simulink model "full_maneuver_single_veh"  (R2020a)
settings: Solver=VariableStepAuto  StartTime=0.0  StopTime=90  FixedStep=0.1  MaxStep=5e-2  RelTol=1e-3
InitFcn:
  | totalVehicles = 5;
  | if exist('vehStatesBus', 'var')==0
  | load vehBuses
  | end
  | if exist('vehErrorsBus', 'var')==0
  | load vehBuses
  | end
libraries: simulink x69, powerlib_meascontrol x6, autolibshared x6, dspsigops x3, eeGeneralControl x2
(part 3 of 6)

== system full_maneuver_single_veh/Fo/Regular Vehicle Following ==
  ego : Inport
  leader : Inport  Port=2
  leaderChange : Inport  Port=3
  extraSpaceFlag : Inport  Port=4
  Bus Selector : BusSelector  OutputSignals=u
  Compute Errors : Subsystem
  Constant : Constant  Value=0
  Define Desired Distance : Subsystem
  NOT : Logic  Operator=NOT  IconShape=distinctive  AllPortsSameDT=off  OutDataTypeStr=boolean
  Rate Limiter : RateLimiter  RisingSlewLimit=maxJerk  FallingSlewLimit=minJerk  SampleTimeMode=inherited
  Rate Limiter1 : RateLimiter  RisingSlewLimit=maxComfJerk  FallingSlewLimit=minComfJerk  SampleTimeMode=inherited
  Switch : Switch  Criteria=u2 > Threshold
  Switch1 : Switch  Criteria=u2 > Threshold
  Veh Following : Subsystem  TreatAsAtomicUnit=on
  Velocity Control : Subsystem  TreatAsAtomicUnit=on
  Velocity Error : Subsystem
  comf saturation : Saturate  UpperLimit=maxComfAccel  LowerLimit=minComfAccel
  errorScope : Scope
  freeFlowVel : Constant  Value=freeFlowVel
  safe saturation : Saturate  UpperLimit=maxAcceleration  LowerLimit=minAcceleration
  switch : Subsystem
  veh foll state : Scope  NumInputPorts=2
  u : Outport  VectorParamsAs1DForOutWhenUnconnected=off
  errors : Outport  Port=2  VectorParamsAs1DForOutWhenUnconnected=off
  gap : Outport  Port=3  VectorParamsAs1DForOutWhenUnconnected=off
  leaderInRange : Outport  Port=4  VectorParamsAs1DForOutWhenUnconnected=off
  wires:
  NOT/1 -> Velocity Error/3(inRange)
  Velocity Error/1(ev) -> Velocity Control/1(ev)
  Velocity Error/2(ea) -> Velocity Control/2(ea)
  leaderChange/1 -> Veh Following/4(leaderChange)
  Veh Following/1(u) -> Switch/1
  Constant/1 -> Compute Errors/5(velFilterReset)
  leader/1 -> Compute Errors/2(leader)
  switch/1(inRange) -> veh foll state/1, Switch/2, leaderInRange/1, Veh Following/5(inRange), NOT/1
  Compute Errors/1(errors) -> switch/1(errors), Veh Following/1(errors), errors/1, errorScope/1
  comf saturation/1 -> Rate Limiter1/1
  safe saturation/1 -> Rate Limiter/1
  Rate Limiter/1 -> Switch1/1  "sat(u)"
  Switch1/1 -> u/1
  Switch/1 -> veh foll state/2, safe saturation/1, comf saturation/1
  Rate Limiter1/1 -> Switch1/3  "sat(u)"
  Compute Errors/3("gap ") -> gap/1, switch/3(gap)
  ego/1 -> Compute Errors/1(ego), Bus Selector/1, Velocity Error/1(ego)
  Velocity Control/1(u) -> Switch/3
  freeFlowVel/1 -> Velocity Error/2(velRef), switch/6(vRef)
  Compute Errors/4(unsafeFlag) -> Switch1/2
  Bus Selector/1 -> Veh Following/3(realInput), Velocity Control/3(realInput)  "<u>"
  Compute Errors/2(errorsDot) -> switch/2(errorsDot), Veh Following/2(errorsDot)
  extraSpaceFlag/1 -> Define Desired Distance/1(extraSpaceFlag)
  Define Desired Distance/1(h) -> Compute Errors/3(h), switch/4(h)
  Define Desired Distance/2(d0) -> Compute Errors/4(d0), switch/5(d0)

== system full_maneuver_single_veh/Fo/findLeader ==
  ego : Inport
  all : Inport  Port=2
  lcFlag : Inport  Port=3
  state : Inport  Port=4
  Compare To Constant : simulink/Logic and Bit Operations/Compare To Constant  relop=~=  const=4  OutDataTypeStr=boolean
  Detect Change : simulink/Logic and Bit Operations/Detect Change  vinit=0  OutDataTypeStr=boolean
  NOT : Logic  Operator=NOT  IconShape=distinctive  AllPortsSameDT=off  OutDataTypeStr=boolean
  OR : Logic  Operator=OR  IconShape=distinctive  AllPortsSameDT=off  OutDataTypeStr=boolean
  Selector : Selector  InputPortWidth=totalVehicles+1  IndexOptions=Index vector (port)  Indices=[1]  OutputSizes=1
  Subsystem : Subsystem
  Vector Concatenate : Concatenate
  farAwayVeh : Subsystem
  realLeaderIdx : Scope
  leader : Outport  VectorParamsAs1DForOutWhenUnconnected=off
  leaderChange : Outport  Port=2  InitialOutput=1  VectorParamsAs1DForOutWhenUnconnected=off
  wires:
  Compare To Constant/1 -> OR/2
  state/1 -> Compare To Constant/1
  ego/1 -> farAwayVeh/1(ego), Subsystem/1(ego)
  all/1 -> Vector Concatenate/1, Subsystem/2(all)
  Subsystem/1(idx) -> realLeaderIdx/1, Selector/2, Detect Change/1
  OR/1 -> Subsystem/Enable
  lcFlag/1 -> NOT/1
  NOT/1 -> OR/1
  Selector/1 -> leader/1
  farAwayVeh/1(Out1) -> Vector Concatenate/2
  Vector Concatenate/1 -> Selector/1
  Detect Change/1 -> leaderChange/1

== system full_maneuver_single_veh/Fo/states routing ==
  delta : Inport
  Info : Inport  Port=2
  u : Inport  Port=3
  Bus Creator : BusCreator  Inputs=7  OutDataTypeStr=Bus: vehStatesBus  NonVirtualBus=on
      settings: InheritFromInputs=off
  Bus Selector : BusSelector  OutputSignals=BdyFrm.Cg.Vel.ydot,BdyFrm.Cg.AngVel.r,InertFrm.RearAxl.Disp.X,InertFrm.Cg.Disp.Y,InertFrm.RearAxl.Vel.Xdot,BdyFrm.Cg.Acc.xddot,InertFrm.Cg.Ang.psi
  Mux : Mux
  latStates : Outport
  observedStates : Outport  Port=2
  wires:
  Bus Creator/1 -> observedStates/1
  Bus Selector/2 -> Mux/4  "<r>"
  Bus Selector/1 -> Mux/2  "<ydot>"
  Mux/1 -> latStates/1
  delta/1 -> Bus Creator/7
  u/1 -> Bus Creator/6  "u"
  Bus Selector/7 -> Mux/3, Bus Creator/5  "<psi>"
  Bus Selector/6 -> Bus Creator/4  "<xddot>"
  Bus Selector/5 -> Bus Creator/3  "<Xdot>"
  Bus Selector/4 -> Mux/1, Bus Creator/2  "<Y>"
  Bus Selector/3 -> Bus Creator/1  "<X>"
  Info/1 -> Bus Selector/1

== system full_maneuver_single_veh/Ld/Regular Vehicle Following ==
  ego : Inport
  leader : Inport  Port=2
  leaderChange : Inport  Port=3
  extraSpaceFlag : Inport  Port=4
  Bus Selector : BusSelector  OutputSignals=u
  Compute Errors : Subsystem
  Constant : Constant  Value=0
  Define Desired Distance : Subsystem
  NOT : Logic  Operator=NOT  IconShape=distinctive  AllPortsSameDT=off  OutDataTypeStr=boolean
  Rate Limiter : RateLimiter  RisingSlewLimit=maxJerk  FallingSlewLimit=minJerk  SampleTimeMode=inherited
  Rate Limiter1 : RateLimiter  RisingSlewLimit=maxComfJerk  FallingSlewLimit=minComfJerk  SampleTimeMode=inherited
  Switch : Switch  Criteria=u2 > Threshold
  Switch1 : Switch  Criteria=u2 > Threshold
  Veh Following : Subsystem  TreatAsAtomicUnit=on
  Velocity Control : Subsystem  TreatAsAtomicUnit=on
  Velocity Error : Subsystem
  comf saturation : Saturate  UpperLimit=maxComfAccel  LowerLimit=minComfAccel
  errorScope : Scope
  freeFlowVel : Constant  Value=freeFlowVel
  safe saturation : Saturate  UpperLimit=maxAcceleration  LowerLimit=minAcceleration
  switch : Subsystem
  veh foll state : Scope  NumInputPorts=2
  u : Outport  VectorParamsAs1DForOutWhenUnconnected=off
  errors : Outport  Port=2  VectorParamsAs1DForOutWhenUnconnected=off
  gap : Outport  Port=3  VectorParamsAs1DForOutWhenUnconnected=off
  leaderInRange : Outport  Port=4  VectorParamsAs1DForOutWhenUnconnected=off
  wires:
  NOT/1 -> Velocity Error/3(inRange)
  Velocity Error/1(ev) -> Velocity Control/1(ev)
  Velocity Error/2(ea) -> Velocity Control/2(ea)
  leaderChange/1 -> Veh Following/4(leaderChange)
  Veh Following/1(u) -> Switch/1
  Constant/1 -> Compute Errors/5(velFilterReset)
  leader/1 -> Compute Errors/2(leader)
  switch/1(inRange) -> veh foll state/1, Switch/2, leaderInRange/1, Veh Following/5(inRange), NOT/1
  Compute Errors/1(errors) -> switch/1(errors), Veh Following/1(errors), errors/1, errorScope/1
  comf saturation/1 -> Rate Limiter1/1
  safe saturation/1 -> Rate Limiter/1
  Rate Limiter/1 -> Switch1/1  "sat(u)"
  Switch1/1 -> u/1
  Switch/1 -> veh foll state/2, safe saturation/1, comf saturation/1
  Rate Limiter1/1 -> Switch1/3  "sat(u)"
  Compute Errors/3("gap ") -> gap/1, switch/3(gap)
  ego/1 -> Compute Errors/1(ego), Bus Selector/1, Velocity Error/1(ego)
  Velocity Control/1(u) -> Switch/3
  freeFlowVel/1 -> Velocity Error/2(velRef), switch/6(vRef)
  Compute Errors/4(unsafeFlag) -> Switch1/2
  Bus Selector/1 -> Veh Following/3(realInput), Velocity Control/3(realInput)  "<u>"
  Compute Errors/2(errorsDot) -> switch/2(errorsDot), Veh Following/2(errorsDot)
  extraSpaceFlag/1 -> Define Desired Distance/1(extraSpaceFlag)
  Define Desired Distance/1(h) -> Compute Errors/3(h), switch/4(h)
  Define Desired Distance/2(d0) -> Compute Errors/4(d0), switch/5(d0)

== system full_maneuver_single_veh/Ld/findLeader ==
  ego : Inport
  all : Inport  Port=2
  lcFlag : Inport  Port=3
  state : Inport  Port=4
  Compare To Constant : simulink/Logic and Bit Operations/Compare To Constant  relop=~=  const=4  OutDataTypeStr=boolean
  Detect Change : simulink/Logic and Bit Operations/Detect Change  vinit=0  OutDataTypeStr=boolean
  NOT : Logic  Operator=NOT  IconShape=distinctive  AllPortsSameDT=off  OutDataTypeStr=boolean
  OR : Logic  Operator=OR  IconShape=distinctive  AllPortsSameDT=off  OutDataTypeStr=boolean
  Selector : Selector  InputPortWidth=totalVehicles+1  IndexOptions=Index vector (port)  Indices=[1]  OutputSizes=1
  Subsystem : Subsystem
  Vector Concatenate : Concatenate
  farAwayVeh : Subsystem
  realLeaderIdx : Scope
  leader : Outport  VectorParamsAs1DForOutWhenUnconnected=off
  leaderChange : Outport  Port=2  InitialOutput=1  VectorParamsAs1DForOutWhenUnconnected=off
  wires:
  Compare To Constant/1 -> OR/2
  state/1 -> Compare To Constant/1
  ego/1 -> farAwayVeh/1(ego), Subsystem/1(ego)
  all/1 -> Vector Concatenate/1, Subsystem/2(all)
  Subsystem/1(idx) -> realLeaderIdx/1, Selector/2, Detect Change/1
  OR/1 -> Subsystem/Enable
  lcFlag/1 -> NOT/1
  NOT/1 -> OR/1
  Selector/1 -> leader/1
  farAwayVeh/1(Out1) -> Vector Concatenate/2
  Vector Concatenate/1 -> Selector/1
  Detect Change/1 -> leaderChange/1

== system full_maneuver_single_veh/Ld/states routing ==
  delta : Inport
  Info : Inport  Port=2
  u : Inport  Port=3
  Bus Creator : BusCreator  Inputs=7  OutDataTypeStr=Bus: vehStatesBus  NonVirtualBus=on
      settings: InheritFromInputs=off
  Bus Selector : BusSelector  OutputSignals=BdyFrm.Cg.Vel.ydot,BdyFrm.Cg.AngVel.r,InertFrm.RearAxl.Disp.X,InertFrm.Cg.Disp.Y,InertFrm.RearAxl.Vel.Xdot,BdyFrm.Cg.Acc.xddot,InertFrm.Cg.Ang.psi
  Mux : Mux
  latStates : Outport
  observedStates : Outport  Port=2
  wires:
  Bus Creator/1 -> observedStates/1
  Bus Selector/2 -> Mux/4  "<r>"
  Bus Selector/1 -> Mux/2  "<ydot>"
  Mux/1 -> latStates/1
  delta/1 -> Bus Creator/7
  u/1 -> Bus Creator/6  "u"
  Bus Selector/7 -> Mux/3, Bus Creator/5  "<psi>"
  Bus Selector/6 -> Bus Creator/4  "<xddot>"
  Bus Selector/5 -> Bus Creator/3  "<Xdot>"
  Bus Selector/4 -> Mux/1, Bus Creator/2  "<Y>"
  Bus Selector/3 -> Bus Creator/1  "<X>"
  Info/1 -> Bus Selector/1

== system full_maneuver_single_veh/Lo/Regular Vehicle Following ==
  ego : Inport
  leader : Inport  Port=2
  leaderChange : Inport  Port=3
  extraSpaceFlag : Inport  Port=4
  Bus Selector : BusSelector  OutputSignals=u
  Compute Errors : Subsystem
  Constant : Constant  Value=0
  Define Desired Distance : Subsystem
  NOT : Logic  Operator=NOT  IconShape=distinctive  AllPortsSameDT=off  OutDataTypeStr=boolean
  Rate Limiter : RateLimiter  RisingSlewLimit=maxJerk  FallingSlewLimit=minJerk  SampleTimeMode=inherited
  Rate Limiter1 : RateLimiter  RisingSlewLimit=maxComfJerk  FallingSlewLimit=minComfJerk  SampleTimeMode=inherited
  Switch : Switch  Criteria=u2 > Threshold
  Switch1 : Switch  Criteria=u2 > Threshold
  Veh Following : Subsystem  TreatAsAtomicUnit=on
  Velocity Control : Subsystem  TreatAsAtomicUnit=on
  Velocity Error : Subsystem
  comf saturation : Saturate  UpperLimit=maxComfAccel  LowerLimit=minComfAccel
  errorScope : Scope
  freeFlowVel : Constant  Value=freeFlowVel
  safe saturation : Saturate  UpperLimit=maxAcceleration  LowerLimit=minAcceleration
  switch : Subsystem
  veh foll state : Scope  NumInputPorts=2
  u : Outport  VectorParamsAs1DForOutWhenUnconnected=off
  errors : Outport  Port=2  VectorParamsAs1DForOutWhenUnconnected=off
  gap : Outport  Port=3  VectorParamsAs1DForOutWhenUnconnected=off
  leaderInRange : Outport  Port=4  VectorParamsAs1DForOutWhenUnconnected=off
  wires:
  Define Desired Distance/2(d0) -> switch/5(d0), Compute Errors/4(d0)
  Define Desired Distance/1(h) -> switch/4(h), Compute Errors/3(h)
  extraSpaceFlag/1 -> Define Desired Distance/1(extraSpaceFlag)
  Compute Errors/2(errorsDot) -> Veh Following/2(errorsDot), switch/2(errorsDot)
  Bus Selector/1 -> Velocity Control/3(realInput), Veh Following/3(realInput)  "<u>"
  Compute Errors/4(unsafeFlag) -> Switch1/2
  freeFlowVel/1 -> switch/6(vRef), Velocity Error/2(velRef)
  Velocity Control/1(u) -> Switch/3
  ego/1 -> Velocity Error/1(ego), Bus Selector/1, Compute Errors/1(ego)
  Compute Errors/3("gap ") -> switch/3(gap), gap/1
  Rate Limiter1/1 -> Switch1/3  "sat(u)"
  Switch/1 -> comf saturation/1, safe saturation/1, veh foll state/2
  Switch1/1 -> u/1
  Rate Limiter/1 -> Switch1/1  "sat(u)"
  safe saturation/1 -> Rate Limiter/1
  comf saturation/1 -> Rate Limiter1/1
  Compute Errors/1(errors) -> errorScope/1, errors/1, Veh Following/1(errors), switch/1(errors)
  switch/1(inRange) -> NOT/1, Veh Following/5(inRange), leaderInRange/1, Switch/2, veh foll state/1
  leader/1 -> Compute Errors/2(leader)
  Constant/1 -> Compute Errors/5(velFilterReset)
  Veh Following/1(u) -> Switch/1
  leaderChange/1 -> Veh Following/4(leaderChange)
  Velocity Error/2(ea) -> Velocity Control/2(ea)
  Velocity Error/1(ev) -> Velocity Control/1(ev)
  NOT/1 -> Velocity Error/3(inRange)

== system full_maneuver_single_veh/Lo/findLeader ==
  ego : Inport
  all : Inport  Port=2
  lcFlag : Inport  Port=3
  state : Inport  Port=4
  Compare To Constant : simulink/Logic and Bit Operations/Compare To Constant  relop=~=  const=4  OutDataTypeStr=boolean
  Detect Change : simulink/Logic and Bit Operations/Detect Change  vinit=0  OutDataTypeStr=boolean
  NOT : Logic  Operator=NOT  IconShape=distinctive  AllPortsSameDT=off  OutDataTypeStr=boolean
  OR : Logic  Operator=OR  IconShape=distinctive  AllPortsSameDT=off  OutDataTypeStr=boolean
  Selector : Selector  InputPortWidth=totalVehicles+1  IndexOptions=Index vector (port)  Indices=[1]  OutputSizes=1
  Subsystem : Subsystem
  Vector Concatenate : Concatenate
  farAwayVeh : Subsystem
  realLeaderIdx : Scope
  leader : Outport  VectorParamsAs1DForOutWhenUnconnected=off
  leaderChange : Outport  Port=2  InitialOutput=1  VectorParamsAs1DForOutWhenUnconnected=off
  wires:
  Detect Change/1 -> leaderChange/1
  Vector Concatenate/1 -> Selector/1
  farAwayVeh/1(Out1) -> Vector Concatenate/2
  Selector/1 -> leader/1
  NOT/1 -> OR/1
  lcFlag/1 -> NOT/1
  OR/1 -> Subsystem/Enable
  Subsystem/1(idx) -> Detect Change/1, Selector/2, realLeaderIdx/1
  all/1 -> Subsystem/2(all), Vector Concatenate/1
  ego/1 -> Subsystem/1(ego), farAwayVeh/1(ego)
  state/1 -> Compare To Constant/1
  Compare To Constant/1 -> OR/2

== system full_maneuver_single_veh/Lo/states routing ==
  delta : Inport
  Info : Inport  Port=2
  u : Inport  Port=3
  Bus Creator : BusCreator  Inputs=7  OutDataTypeStr=Bus: vehStatesBus  NonVirtualBus=on
      settings: InheritFromInputs=off
  Bus Selector : BusSelector  OutputSignals=BdyFrm.Cg.Vel.ydot,BdyFrm.Cg.AngVel.r,InertFrm.RearAxl.Disp.X,InertFrm.Cg.Disp.Y,InertFrm.RearAxl.Vel.Xdot,BdyFrm.Cg.Acc.xddot,InertFrm.Cg.Ang.psi
  Mux : Mux
  latStates : Outport
  observedStates : Outport  Port=2
  wires:
  Info/1 -> Bus Selector/1
  Bus Selector/3 -> Bus Creator/1  "<X>"
  Bus Selector/4 -> Bus Creator/2, Mux/1  "<Y>"
  Bus Selector/5 -> Bus Creator/3  "<Xdot>"
  Bus Selector/6 -> Bus Creator/4  "<xddot>"
  Bus Selector/7 -> Bus Creator/5, Mux/3  "<psi>"
  u/1 -> Bus Creator/6  "u"
  delta/1 -> Bus Creator/7
  Mux/1 -> latStates/1
  Bus Selector/1 -> Mux/2  "<ydot>"
  Bus Selector/2 -> Mux/4  "<r>"
  Bus Creator/1 -> observedStates/1

== system full_maneuver_single_veh/p1/Error to Follower ==
  ego : Inport
  follower : Inport  Port=2
  Bus Selector : BusSelector  OutputSignals=X,Xdot
  Bus Selector1 : BusSelector  OutputSignals=X,Xdot
  Multiply : Product
  Mux : Mux  Inputs=2
  Sum : Sum  Inputs=-+|
  Sum1 : Sum  Inputs=++|
  Sum2 : Sum  Inputs=+-|
  Sum3 : Sum  Inputs=|++
  Sum4 : Sum  Inputs=-+|
  d0 : Constant  Value=d0
  h : Constant  Value=h
  vLen : Constant  Value=lr+lf
  errors : Outport  VectorParamsAs1DForOutWhenUnconnected=off
  wires:
  Mux/1 -> errors/1
  Sum4/1 -> Mux/2
  Bus Selector1/2 -> Sum4/2  "<Xdot>"
  Bus Selector/2 -> Multiply/1, Sum4/1  "<Xdot>"
  ego/1 -> Bus Selector1/1
  follower/1 -> Bus Selector/1
  vLen/1 -> Sum1/1
  Multiply/1 -> Sum3/1
  Sum/1 -> Sum2/1  "gap"
  Bus Selector/1 -> Sum1/2  "<X>"
  Sum3/1 -> Sum2/2  "desired  gap"
  Sum1/1 -> Sum/1  "x (front bumber)"
  Bus Selector1/1 -> Sum/2  "<X>"
  Sum2/1 -> Mux/1
  h/1 -> Multiply/2  "time headway"
  d0/1 -> Sum3/2  "gap at  standstill"

== system full_maneuver_single_veh/p1/Find Leader ==
  ego : Inport
  all : Inport  Port=2
  lcFlag : Inport  Port=3
  state : Inport  Port=4
  Compare To Constant : simulink/Logic and Bit Operations/Compare To Constant  relop=~=  const=4  OutDataTypeStr=boolean
  Detect Change : simulink/Logic and Bit Operations/Detect Change  vinit=0  OutDataTypeStr=boolean
  NOT : Logic  Operator=NOT  IconShape=distinctive  AllPortsSameDT=off  OutDataTypeStr=boolean
  OR : Logic  Operator=OR  IconShape=distinctive  AllPortsSameDT=off  OutDataTypeStr=boolean
  Selector : Selector  InputPortWidth=totalVehicles+1  IndexOptions=Index vector (port)  Indices=[1]  OutputSizes=1
  Subsystem : Subsystem
  Vector Concatenate : Concatenate
  farAwayVeh : Subsystem
  realLeaderIdx : Scope
  leader : Outport  VectorParamsAs1DForOutWhenUnconnected=off
  leaderChange : Outport  Port=2  InitialOutput=1  VectorParamsAs1DForOutWhenUnconnected=off
  wires:
  Detect Change/1 -> leaderChange/1
  Vector Concatenate/1 -> Selector/1
  farAwayVeh/1(Out1) -> Vector Concatenate/2
  Selector/1 -> leader/1
  NOT/1 -> OR/1
  lcFlag/1 -> NOT/1
  OR/1 -> Subsystem/Enable
  Subsystem/1(idx) -> Detect Change/1, Selector/2, realLeaderIdx/1
  all/1 -> Subsystem/2(all), Vector Concatenate/1
  ego/1 -> farAwayVeh/1(ego), Subsystem/1(ego)
  state/1 -> Compare To Constant/1
  Compare To Constant/1 -> OR/2

== system full_maneuver_single_veh/p1/Lateral Control ==
  measuredStates : Inport
  yRef : Inport  Port=2
  Enable : EnablePort
  Demux2 : Demux
  Full State Observer : Subsystem  Commented=on
  Gain : Gain  Gain=5
  Gain1 : Gain  Gain=Klat  Multiplication=Matrix(K*u)
  Integrator : Integrator  InitialCondition=y0
  Pad : dspsigops/Pad  padAlong=Columns  dimsToPad=1  valSrc=Specify via dialog  padVal=0  spec=Output size  padNumOutRowsSpecMethod=User-specified  numOutRows=4  padNumOutColsSpecMethod=User-specified  numOutCols=1  isVarDimsMode=off  padBeginning=0  padEnd=0  outSizeMode=User-specified  outSize=1  padSigAt=End  trunc_flag=None  roundingMode=Floor  overflowMode=off  truncOrWrapMode=Truncate  wrap_flag=None
      settings: SourceProductBaseCode=DS
  Rate Limiter : RateLimiter  RisingSlewLimit=maxDeltaDot  FallingSlewLimit=-maxDeltaDot  SampleTimeMode=inherited
  Saturation : Saturate  UpperLimit=maxDelta  LowerLimit=-maxDelta
  Saturation1 : Saturate  UpperLimit=2  LowerLimit=-2
  Scope : Scope  NumInputPorts=4
  Scope1 : Scope  NumInputPorts=2
  Selector : Selector  InputPortWidth=4  IndexOptions=Index vector (dialog)  Indices=[1]  OutputSizes=1
  Sum : Sum  Inputs=|+-
  Sum2 : Sum  Inputs=|+-
  delta : Outport  VectorParamsAs1DForOutWhenUnconnected=off
  ey : Outport  Port=2  VectorParamsAs1DForOutWhenUnconnected=off
  vy_hat : Outport  Port=3  InitialOutput=0.3  VectorParamsAs1DForOutWhenUnconnected=off
  wires:
  Rate Limiter/1 -> Full State Observer/2(delta), Scope1/1, delta/1  "delta"
  Demux2/1 -> Scope/1
  Integrator/1 -> Sum2/2, Pad/1
  Gain1/1 -> Scope1/2, Saturation/1
  Sum/1 -> Selector/1, Gain1/1
  Pad/1 -> Sum/1
  Demux2/4 -> Scope/4
  Demux2/2 -> vy_hat/1, Scope/2
  Sum2/1 -> Gain/1
  Saturation/1 -> Rate Limiter/1
  Demux2/3 -> Scope/3
  yRef/1 -> Sum2/1
  measuredStates/1 -> Full State Observer/1(measuredOutputs), Demux2/1, Sum/2  "estStates"
  Gain/1 -> Saturation1/1
  Saturation1/1 -> Integrator/1
  Selector/1 -> ey/1

== system full_maneuver_single_veh/p1/Maneuver State ==
  note: States are:
      | 0 - Lane keeping
      | 1 - Longitudinal Adjustment
      | 2 - Steady State
      | 3 - Safe to LC
      | 4 - Performing LC
      | 5 - LC is done
      | 6 - Long Adj done
  u : Inport
  errors : Inport  Port=2
  virtualErrors : Inport  Port=3
  followerErrors : Inport  Port=4
  canStartLC : Inport  Port=5
  extraSpace : Inport  Port=6
  lcDone : Inport  Port=7
  Enable : EnablePort
  AND : Logic  IconShape=distinctive  AllPortsSameDT=off  OutDataTypeStr=boolean
  AND1 : Logic  IconShape=distinctive  AllPortsSameDT=off  OutDataTypeStr=boolean
  AND2 : Logic  Inputs=3  IconShape=distinctive  AllPortsSameDT=off  OutDataTypeStr=boolean
  AND{3..7} (5 alike) : Logic  IconShape=distinctive  AllPortsSameDT=off  OutDataTypeStr=fixdt(1,16)
  Constant : Constant
  Data Type Conversion : DataTypeConversion  OutMin=0  OutMax=1  OutDataTypeStr=fixdt(1,16)
  Memory : Memory
  NOT1 : Logic  Operator=NOT  IconShape=distinctive  AllPortsSameDT=off  OutDataTypeStr=boolean
  On Delay : powerlib_meascontrol/Logic/On Delay  DelayType=On delay  delay=1  ic=0  Ts=0
  On Delay1 : powerlib_meascontrol/Logic/On Delay  DelayType=On delay  delay=0.2  ic=0  Ts=0
  Scope : Scope  NumInputPorts=5
  Sum : Sum  Inputs=++++++
  Triggered Subsystem : Subsystem  TreatAsAtomicUnit=on
  Triggered Subsystem1 : Subsystem  TreatAsAtomicUnit=on
  safeErrors : Subsystem
  safeErrors1 : Subsystem
  safeErrors2 : Subsystem
  steadyState : Subsystem
  state : Outport  InitialOutput=0  VectorParamsAs1DForOutWhenUnconnected=off
  wires:
  Memory/1 -> AND3/2
  AND4/1 -> AND5/1, Scope/2, Sum/3
  safeErrors/1(safetyFlag) -> AND4/2
  Sum/1 -> state/1
  AND3/1 -> AND4/1, Scope/1, Sum/2
  AND5/1 -> AND6/1, Scope/3, Sum/4
  Constant/1 -> Data Type Conversion/1, AND3/1
  AND6/1 -> Scope/4, Sum/5, AND7/1
  AND/1 -> AND7/2
  Data Type Conversion/1 -> Sum/1
  AND7/1 -> Triggered Subsystem/Trigger, Scope/5
  lcDone/1 -> AND6/2
  canStartLC/1 -> AND5/2
  Triggered Subsystem/1(Out1) -> Sum/6
  virtualErrors/1 -> safeErrors2/1(errors)
  errors/1 -> safeErrors1/1(errors)
  followerErrors/1 -> safeErrors/1(errors)
  On Delay1/1 -> AND/2
  AND2/1 -> Triggered Subsystem1/Trigger
  safeErrors1/1(safetyFlag) -> AND1/2
  extraSpace/1 -> NOT1/1, On Delay/1
  On Delay/1 -> AND2/3
  NOT1/1 -> On Delay1/1
  Triggered Subsystem1/1(Out1) -> Memory/1
  safeErrors2/1(safetyFlag) -> AND2/2
  steadyState/1(ssFlag) -> AND1/1
  AND1/1 -> AND2/1, AND/1  "steady state"
  u/1 -> steadyState/1(u)

== system full_maneuver_single_veh/p1/Platoon Gap Generation Management ==
  posInPlatoon : Inport
  strategy : Inport  Port=2
  platoonState : Inport  Port=3
  Enable : EnablePort
  Scope : Scope  NumInputPorts=2
  assignExtraSpace : MATLAB Function  TreatAsAtomicUnit=on
  assignvirtualLeader : MATLAB Function  TreatAsAtomicUnit=on
  assignVL : Outport  VectorParamsAs1DForOutWhenUnconnected=off
  extraSpace : Outport  Port=2  VectorParamsAs1DForOutWhenUnconnected=off
  wires:
  assignExtraSpace/1(extraSpaceFlag) -> Scope/2, extraSpace/1
  strategy/1 -> assignvirtualLeader/1(strategy), assignExtraSpace/1(strategy)
  posInPlatoon/1 -> assignvirtualLeader/2(posInPlatoon), assignExtraSpace/2(posInPlatoon)
  platoonState/1 -> assignvirtualLeader/3(platoonState), assignExtraSpace/3(platoonState)
  assignvirtualLeader/1(virtualLeaderFlag) -> Scope/1, assignVL/1

== system full_maneuver_single_veh/p1/Platoon LC Management ==
  platoonStates : Inport
  strategy : Inport  Port=2
  Compare To Constant : simulink/Logic and Bit Operations/Compare To Constant  relop=>  const=1  OutDataTypeStr=boolean
  Compare To Constant1 : simulink/Logic and Bit Operations/Compare To Constant  relop=>  const=2  OutDataTypeStr=boolean
  OR : Logic  Operator=OR  IconShape=distinctive  AllPortsSameDT=off  OutDataTypeStr=boolean
  Selector : Selector  IndexOptions=Index vector (port)  Indices=[1 3]  OutputSizes=1
  Width : Width
  Out1 : Outport  VectorParamsAs1DForOutWhenUnconnected=off
  wires:
  strategy/1 -> Compare To Constant/1
  Compare To Constant/1 -> OR/2
  OR/1 -> Out1/1
  platoonStates/1 -> Width/1, Selector/1
  Width/1 -> Selector/2
  Selector/1 -> Compare To Constant1/1
  Compare To Constant1/1 -> OR/1

== system full_maneuver_single_veh/p1/Regular Vehicle Following ==
  ego : Inport
  leader : Inport  Port=2
  leaderChange : Inport  Port=3
  extraSpaceFlag : Inport  Port=4
  Bus Selector : BusSelector  OutputSignals=u
  Compute Errors : Subsystem
  Constant : Constant  Value=0
  Define Desired Distance : Subsystem
  Rate Limiter : RateLimiter  RisingSlewLimit=maxJerk  FallingSlewLimit=minJerk  SampleTimeMode=inherited
  Rate Limiter1 : RateLimiter  RisingSlewLimit=maxComfJerk  FallingSlewLimit=minComfJerk  SampleTimeMode=inherited
  Switch : Switch  Criteria=u2 > Threshold
  Switch1 : Switch  Criteria=u2 > Threshold
  Veh Following : Subsystem  TreatAsAtomicUnit=on
  Velocity Control : Subsystem  TreatAsAtomicUnit=on
  Velocity Error : Subsystem
  comf saturation : Saturate  UpperLimit=maxComfAccel  LowerLimit=minComfAccel
  errorScope : Scope
  freeFlowVel : Constant  Value=freeFlowVel
  safe saturation : Saturate  UpperLimit=maxAcceleration  LowerLimit=minAcceleration
  switch free flow : Subsystem
  veh foll state : Scope  NumInputPorts=2
  u : Outport  VectorParamsAs1DForOutWhenUnconnected=off
  errors : Outport  Port=2  VectorParamsAs1DForOutWhenUnconnected=off
  gap : Outport  Port=3  VectorParamsAs1DForOutWhenUnconnected=off
  wires:
  Define Desired Distance/2(d0) -> switch free flow/5(d0), Compute Errors/4(d0)
  Define Desired Distance/1(h) -> switch free flow/4(h), Compute Errors/3(h)
  Compute Errors/2(errorsDot) -> switch free flow/2(errorsDot), Veh Following/2(errorsDot)
  Bus Selector/1 -> Velocity Control/3(realInput), Veh Following/3(realInput)  "<u>"
  Compute Errors/4(unsafeFlag) -> Switch1/2
  freeFlowVel/1 -> switch free flow/6(vRef), Velocity Error/2(velRef)
  Velocity Control/1(u) -> Switch/3
  ego/1 -> Velocity Error/1(ego), Bus Selector/1, Compute Errors/1(ego)
  Compute Errors/3("gap ") -> switch free flow/3(gap), gap/1
  Rate Limiter1/1 -> Switch1/3  "sat(u)"
  Switch/1 -> comf saturation/1, safe saturation/1, veh foll state/2
  Switch1/1 -> u/1
  Rate Limiter/1 -> Switch1/1  "sat(u)"
  safe saturation/1 -> Rate Limiter/1
  comf saturation/1 -> Rate Limiter1/1
  Compute Errors/1(errors) -> errorScope/1, errors/1, Veh Following/1(errors), switch free flow/1(errors)
  leader/1 -> Compute Errors/2(leader)
  Constant/1 -> Compute Errors/5(velFilterReset)
  Veh Following/1(u) -> Switch/1
  leaderChange/1 -> Veh Following/4(leaderChange)
  Velocity Error/2(ea) -> Velocity Control/2(ea)
  Velocity Error/1(ev) -> Velocity Control/1(ev)
  switch free flow/1(inRange) -> Veh Following/5(inRange), veh foll state/1, Switch/2
  extraSpaceFlag/1 -> Velocity Error/3(filterReset), Define Desired Distance/1(extraSpaceFlag)

== system full_maneuver_single_veh/p1/Subsystem ==
  state : Inport
  u : Inport  Port=2
  Compare To Constant : simulink/Logic and Bit Operations/Compare To Constant  relop===  const=7  OutDataTypeStr=boolean
  Scope : Scope
  Switch1 : Switch  Criteria=u2 > Threshold
  comf saturation : Saturate  UpperLimit=maxComfAccel  LowerLimit=minComfAccel
  comf jerk : RateLimiter  RisingSlewLimit=maxComfJerk  FallingSlewLimit=minComfJerk  SampleTimeMode=inherited
  safe saturation : Saturate  UpperLimit=maxAcceleration  LowerLimit=minAcceleration
  safe jerk : RateLimiter  RisingSlewLimit=maxJerk  FallingSlewLimit=minJerk  SampleTimeMode=inherited
  sat(u) : Outport  VectorParamsAs1DForOutWhenUnconnected=off
  wires:
  Compare To Constant/1 -> Switch1/2
  Switch1/1 -> sat(u)/1, Scope/1
  comf jerk/1 -> Switch1/3
  u/1 -> safe saturation/1, comf saturation/1
  state/1 -> Compare To Constant/1
  comf saturation/1 -> comf jerk/1
  safe jerk/1 -> Switch1/1
  safe saturation/1 -> safe jerk/1

== system full_maneuver_single_veh/p1/Triggered Subsystem ==
  Trigger : TriggerPort  VariantControl=Variant
  Constant : Constant
  lcFlag : Outport  InitialOutput=0  VectorParamsAs1DForOutWhenUnconnected=off
  wires:
  Constant/1 -> lcFlag/1

== system full_maneuver_single_veh/p1/Virtual Follower Manager ==
  all : Inport
  posInPlatoon : Inport  Port=2
  lcStrategy : Inport  Port=3
  Enable : EnablePort
  Selector1 : Selector  InputPortWidth=totalVehicles  IndexOptions=Index vector (port)  Indices=[1]  OutputSizes=1
  Width : Width
  determineVirtualFollower : MATLAB Function  TreatAsAtomicUnit=on
  virtualFollower : Outport
  wires:
  Selector1/1 -> virtualFollower/1
  all/1 -> Width/1, Selector1/1
  posInPlatoon/1 -> determineVirtualFollower/2(posInPlatoon)
  determineVirtualFollower/1(virtualFollowerIdx) -> Selector1/2
  lcStrategy/1 -> determineVirtualFollower/3(lcStrategy)
  Width/1 -> determineVirtualFollower/1(nVehicles)

== system full_maneuver_single_veh/p1/Virtual Leader Manager ==
  all : Inport
  lcFlag : Inport  Port=2
  lcDone : Inport  Port=3
  posInPlatoon : Inport  Port=4
  lcStrategy : Inport  Port=5
  Detect Change : simulink/Logic and Bit Operations/Detect Change  vinit=0  OutDataTypeStr=boolean
  Selector : Selector  InputPortWidth=totalVehicles  IndexOptions=Index vector (port)  Indices=[1]  OutputSizes=1
  Width : Width
  determineVirtualLeader : MATLAB Function  TreatAsAtomicUnit=on
  virtualVehs : Scope
  virtualLeader : Outport  VectorParamsAs1DForOutWhenUnconnected=off
  leaderChange : Outport  Port=2  VectorParamsAs1DForOutWhenUnconnected=off
  wires:
  lcStrategy/1 -> determineVirtualLeader/5(lcStrategy)
  posInPlatoon/1 -> determineVirtualLeader/4(posInPlatoon)
  lcDone/1 -> determineVirtualLeader/3(lcDone)
  lcFlag/1 -> determineVirtualLeader/2(lcFlag)
  Width/1 -> determineVirtualLeader/1(nVehicles)
  determineVirtualLeader/1(virtualLeaderIdx) -> virtualVehs/1, Detect Change/1, Selector/2
  Detect Change/1 -> leaderChange/1
  Selector/1 -> virtualLeader/1
  all/1 -> Width/1, Selector/1

== system full_maneuver_single_veh/p1/Virtual Vehicle Following ==
  ego : Inport
  virtualLeader : Inport  Port=2
  leaderChange : Inport  Port=3
  extraSpaceFlag : Inport  Port=4
  Bus Selector : BusSelector  OutputSignals=u
  Compute Errors : Subsystem
  Define Desired Distance : Subsystem
  Min Velocity Control : Subsystem  TreatAsAtomicUnit=on
  Min Velocity Error : Subsystem
  NOT : Logic  Operator=NOT  IconShape=distinctive  AllPortsSameDT=off  OutDataTypeStr=boolean
  Scope : Scope  NumInputPorts=2
  Switch : Switch  Criteria=u2 > Threshold
  Terminator : Terminator
  Virtual Leader Following : Subsystem  TreatAsAtomicUnit=on
  switch min vel : Subsystem
  vMin : Constant  Value=vMin
  u : Outport  InitialOutput=0  VectorParamsAs1DForOutWhenUnconnected=off
  virtualErrors : Outport  Port=2  OutputWhenDisabled=reset  InitialOutput=[0, 0]  VectorParamsAs1DForOutWhenUnconnected=off
  virtualGap : Outport  Port=3  OutputWhenDisabled=reset  InitialOutput=[0]  VectorParamsAs1DForOutWhenUnconnected=off
  wires:
  Define Desired Distance/2(d0) -> Compute Errors/4(d0), switch min vel/5(d0)
  Define Desired Distance/1(h) -> Compute Errors/3(h), switch min vel/4(h)
  Compute Errors/2(errorsDot) -> switch min vel/2(errorsDot), Virtual Leader Following/2(errorsDot)
  Compute Errors/4(unsafeFlag) -> Terminator/1
  leaderChange/1 -> Virtual Leader Following/4(leaderChange), Compute Errors/5(velFilterReset)
  Switch/1 -> u/1, Scope/2
  virtualLeader/1 -> Compute Errors/2(leader)
  Compute Errors/1(errors) -> virtualErrors/1, Virtual Leader Following/1(errors), switch min vel/1(errors)
  vMin/1 -> switch min vel/6(vRef), Min Velocity Error/2(velRef)
  ego/1 -> Bus Selector/1, Min Velocity Error/1(ego), Compute Errors/1(ego)
  Virtual Leader Following/1(u) -> Switch/1  "uVehFoll"
  Compute Errors/3("gap ") -> switch min vel/3(gap), virtualGap/1
  Min Velocity Control/1(u) -> Switch/3  "uMinVelControl"
  extraSpaceFlag/1 -> Define Desired Distance/1(extraSpaceFlag)
  switch min vel/1(inRange) -> Min Velocity Error/3(filterReset), NOT/1
  NOT/1 -> Virtual Leader Following/5(inRange), Scope/1, Switch/2
  Min Velocity Error/1(ev) -> Min Velocity Control/1(ev)
  Min Velocity Error/2(ea) -> Min Velocity Control/2(ea)
  Bus Selector/1 -> Virtual Leader Following/3(realInput), Min Velocity Control/3(realInput)  "<u>"

== system full_maneuver_single_veh/p1/lateral steady state ==
  u : Inport
  AND : Logic  IconShape=distinctive  AllPortsSameDT=off  OutDataTypeStr=boolean
  Abs2 : Abs
  Compare To Constant2 : simulink/Logic and Bit Operations/Compare To Constant  relop=<=  const=0.2  OutDataTypeStr=boolean
  Demux : Demux  Outputs=2
  Mux : Mux  Inputs=2
  Transport Delay2 : TransportDelay
  ssFlag : Outport  VectorParamsAs1DForOutWhenUnconnected=off
  wires:
  Demux/2 -> AND/2
  Mux/1 -> Abs2/1
  Compare To Constant2/1 -> Demux/1
  AND/1 -> ssFlag/1
  Transport Delay2/1 -> Mux/1
  Demux/1 -> AND/1
  Abs2/1 -> Compare To Constant2/1
  u/1 -> Mux/2, Transport Delay2/1

== system full_maneuver_single_veh/p1/states routing ==
  delta : Inport
  Info : Inport  Port=2
  u : Inport  Port=3
  Bus Creator : BusCreator  Inputs=7  OutDataTypeStr=Bus: vehStatesBus  NonVirtualBus=on
      settings: InheritFromInputs=off
  Bus Selector : BusSelector  OutputSignals=BdyFrm.Cg.Vel.ydot,BdyFrm.Cg.AngVel.r,InertFrm.RearAxl.Disp.X,InertFrm.Cg.Disp.Y,InertFrm.RearAxl.Vel.Xdot,BdyFrm.Cg.Acc.xddot,InertFrm.Cg.Ang.psi
  Mux : Mux
  latStates : Outport
  observedStates : Outport  Port=2
  wires:
  Info/1 -> Bus Selector/1
  Bus Selector/3 -> Bus Creator/1  "<X>"
  Bus Selector/4 -> Bus Creator/2, Mux/1  "<Y>"
  Bus Selector/5 -> Bus Creator/3  "<Xdot>"
  Bus Selector/6 -> Bus Creator/4  "<xddot>"
  Bus Selector/7 -> Bus Creator/5, Mux/3  "<psi>"
  u/1 -> Bus Creator/6
  delta/1 -> Bus Creator/7
  Mux/1 -> latStates/1
  Bus Selector/1 -> Mux/2  "<ydot>"
  Bus Selector/2 -> Mux/4  "<r>"
  Bus Creator/1 -> observedStates/1

== system full_maneuver_single_veh/Fd/Find Leader/Subsystem ==
  ego : Inport
  all : Inport  Port=2
  Enable : EnablePort
  MATLAB Function : MATLAB Function  TreatAsAtomicUnit=on
  idx : Outport  InitialOutput=1  VectorParamsAs1DForOutWhenUnconnected=off
  wires:
  all/1 -> MATLAB Function/2(allVehicles)
  MATLAB Function/1(leaderIdx) -> idx/1
  ego/1 -> MATLAB Function/1(ego)

== system full_maneuver_single_veh/Fd/Find Leader/farAwayVeh ==
  ego : Inport  OutDataTypeStr=Bus: vehStatesBus
  Bus Assignment : BusAssignment  AssignedSignals=X
  Bus Selector : BusSelector  OutputSignals=X
  Constant : Constant  Value=1000
  Sum : Sum  Inputs=|++
  Out1 : Outport  OutDataTypeStr=Bus: vehStatesBus  VectorParamsAs1DForOutWhenUnconnected=off
  wires:
  Sum/1 -> Bus Assignment/2  "X"
  Bus Selector/1 -> Sum/1  "<X>"
  Bus Assignment/1 -> Out1/1
  Constant/1 -> Sum/2
  ego/1 -> Bus Selector/1, Bus Assignment/1

== system full_maneuver_single_veh/Fd/Lateral Control/Full State Observer ==
  note: xhat
  note: yhat
  measuredOutputs : Inport
  delta : Inport  Port=2
  Add1 : Sum  Inputs=|-+
  Gain : Gain  Gain=B  Multiplication=Matrix(K*u)
  Gain1 : Gain  Gain=C  Multiplication=Matrix(K*u)
  Gain2 : Gain  Gain=L  Multiplication=Matrix(K*u)
  Gain3 : Gain  Gain=A  Multiplication=Matrix(K*u)
  Integrator : Integrator  InitialCondition=[y0; 0; 0; 0]
  Signal Specification : SignalSpecification  Dimensions=[size(C,1) 1]
  Sum : Sum  Inputs=+++
  xhat : Outport  VectorParamsAs1DForOutWhenUnconnected=off
  wires:
  Add1/1 -> Signal Specification/1
  Integrator/1 -> xhat/1, Gain3/1, Gain1/1
  Gain1/1 -> Add1/1
  Sum/1 -> Integrator/1
  measuredOutputs/1 -> Add1/2
  delta/1 -> Gain/1
  Gain/1 -> Sum/3
  Gain3/1 -> Sum/2
  Signal Specification/1 -> Gain2/1
  Gain2/1 -> Sum/1

== system full_maneuver_single_veh/Fd/Maneuver State/Triggered Subsystem ==
  Trigger : TriggerPort  VariantControl=Variant
  Constant : Constant  OutDataTypeStr=fixdt(1,16,0)
  Out1 : Outport  InitialOutput=0  VectorParamsAs1DForOutWhenUnconnected=off
  wires:
  Constant/1 -> Out1/1

== system full_maneuver_single_veh/Fd/Maneuver State/Triggered Subsystem1 ==
  Trigger : TriggerPort  VariantControl=Variant
  Constant : Constant  Value=true  OutDataTypeStr=boolean
  Out1 : Outport  OutDataTypeStr=boolean  InitialOutput=0  VectorParamsAs1DForOutWhenUnconnected=off
  wires:
  Constant/1 -> Out1/1

== system full_maneuver_single_veh/Fd/Maneuver State/safeErrors ==
  errors : Inport
  AND : Logic  Inputs=1  IconShape=distinctive  AllPortsSameDT=off  OutDataTypeStr=boolean
  Compare To Constant4 : simulink/Logic and Bit Operations/Compare To Constant  relop=>=  const=-0.1  OutDataTypeStr=boolean
  Memory : Memory
  Triggered Subsystem1 : Subsystem  TreatAsAtomicUnit=on
  safetyFlag : Outport  VectorParamsAs1DForOutWhenUnconnected=off
  wires:
  Memory/1 -> safetyFlag/1
  Triggered Subsystem1/1(Out1) -> Memory/1
  errors/1 -> Compare To Constant4/1
  AND/1 -> Triggered Subsystem1/Trigger
  Compare To Constant4/1 -> AND/1

== system full_maneuver_single_veh/Fd/Maneuver State/safeErrors1 ==
  errors : Inport
  AND : Logic  Inputs=1  IconShape=distinctive  AllPortsSameDT=off  OutDataTypeStr=boolean
  Compare To Constant4 : simulink/Logic and Bit Operations/Compare To Constant  relop=>=  const=-0.1  OutDataTypeStr=boolean
  safetyFlag : Outport  VectorParamsAs1DForOutWhenUnconnected=off
  wires:
  AND/1 -> safetyFlag/1
  errors/1 -> Compare To Constant4/1
  Compare To Constant4/1 -> AND/1

== system full_maneuver_single_veh/Fd/Maneuver State/safeErrors2 ==
  errors : Inport
  AND : Logic  Inputs=1  IconShape=distinctive  AllPortsSameDT=off  OutDataTypeStr=boolean
  Compare To Constant4 : simulink/Logic and Bit Operations/Compare To Constant  relop=>=  const=-0.1  OutDataTypeStr=boolean
  safetyFlag : Outport  VectorParamsAs1DForOutWhenUnconnected=off
  wires:
  errors/1 -> Compare To Constant4/1
  AND/1 -> safetyFlag/1
  Compare To Constant4/1 -> AND/1

== system full_maneuver_single_veh/Fd/Maneuver State/steadyState ==
  u : Inport
  AND : Logic  Inputs=1  IconShape=distinctive  AllPortsSameDT=off  OutDataTypeStr=boolean
  Abs2 : Abs
  Compare To Constant2 : simulink/Logic and Bit Operations/Compare To Constant  relop=<=  const=0.2  OutDataTypeStr=boolean
  Mux : Mux  Inputs=2
  Transport Delay2 : TransportDelay
  ssFlag : Outport  VectorParamsAs1DForOutWhenUnconnected=off
  wires:
  Mux/1 -> Abs2/1
  AND/1 -> ssFlag/1
  Transport Delay2/1 -> Mux/1
  Abs2/1 -> Compare To Constant2/1
  u/1 -> Mux/2, Transport Delay2/1
  Compare To Constant2/1 -> AND/1

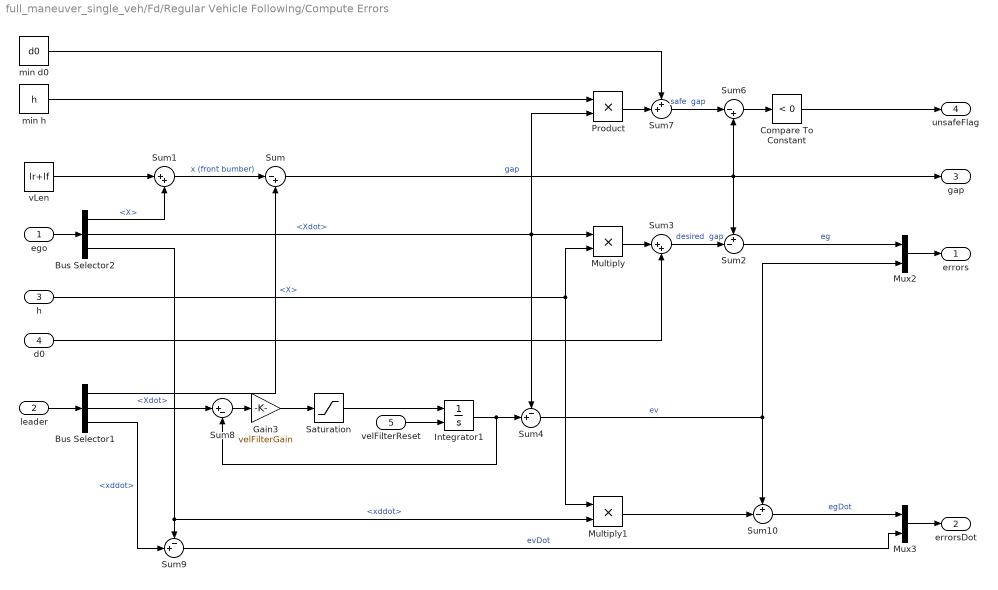
== system full_maneuver_single_veh/Fd/Regular Vehicle Following/Compute Errors ==
  ego : Inport
  leader : Inport  Port=2
  h : Inport  Port=3
  d0 : Inport  Port=4
  velFilterReset : Inport  Port=5
  Bus Selector1 : BusSelector  OutputSignals=X,Xdot,xddot
  Bus Selector2 : BusSelector  OutputSignals=X,Xdot,xddot
  Compare To Constant : simulink/Logic and Bit Operations/Compare To Constant  relop=<  const=0  OutDataTypeStr=boolean
  Gain3 : Gain  Gain=velFilterGain
  Integrator1 : Integrator  ExternalReset=rising  InitialCondition=vx0
  Multiply : Product
  Multiply1 : Product
  Mux2 : Mux  Inputs=2
  Mux3 : Mux  Inputs=2
  Product : Product
  Saturation : Saturate  UpperLimit=maxAcceleration  LowerLimit=minAcceleration
  Sum : Sum  Inputs=|-+
  Sum1 : Sum  Inputs=|++
  Sum10 : Sum  Inputs=+-|
  Sum2 : Sum  Inputs=+-|
  Sum3 : Sum  Inputs=|++
  Sum4 : Sum  Inputs=-+|
  Sum6 : Sum  Inputs=|-+
  Sum7 : Sum  Inputs=++|
  Sum8 : Sum  Inputs=|+-
  Sum9 : Sum  Inputs=-+|
  min d0 : Constant  Value=d0
  min h : Constant  Value=h
  vLen : Constant  Value=lr+lf
  errors : Outport  VectorParamsAs1DForOutWhenUnconnected=off
  errorsDot : Outport  Port=2
  "gap " : Outport  Port=3  VectorParamsAs1DForOutWhenUnconnected=off
  unsafeFlag : Outport  Port=4  VectorParamsAs1DForOutWhenUnconnected=off
  wires:
  Mux2/1 -> errors/1
  velFilterReset/1 -> Integrator1/2
  Sum6/1 -> Compare To Constant/1
  Sum7/1 -> Sum6/1  "safe  gap"
  min h/1 -> Product/1
  Compare To Constant/1 -> unsafeFlag/1
  Sum2/1 -> Mux2/1  "eg"
  Bus Selector1/1 -> Sum/2  "<X>"
  Product/1 -> Sum7/2
  Sum3/1 -> Sum2/2  "desired  gap"
  Sum1/1 -> Sum/1  "x (front bumber)"
  Bus Selector2/2 -> Sum4/1, Multiply/1, Product/2  "<Xdot>"
  d0/1 -> Sum3/2
  vLen/1 -> Sum1/1
  min d0/1 -> Sum7/1
  Multiply/1 -> Sum3/1
  Sum/1 -> Sum2/1, Sum6/2, "gap "/1  "gap"
  Bus Selector2/1 -> Sum1/2  "<X>"
  h/1 -> Multiply/2, Multiply1/1
  Bus Selector1/2 -> Sum8/1  "<Xdot>"
  Sum4/1 -> Mux2/2, Sum10/1  "ev"
  Gain3/1 -> Saturation/1
  Saturation/1 -> Integrator1/1
  Integrator1/1 -> Sum4/2, Sum8/2
  Sum8/1 -> Gain3/1
  Bus Selector1/3 -> Sum9/2  "<xddot>"
  Bus Selector2/3 -> Sum9/1, Multiply1/2  "<xddot>"
  Multiply1/1 -> Sum10/2
  Sum10/1 -> Mux3/1  "egDot"
  Sum9/1 -> Mux3/2  "evDot"
  Mux3/1 -> errorsDot/1
  ego/1 -> Bus Selector2/1
  leader/1 -> Bus Selector1/1

== system full_maneuver_single_veh/Fd/Regular Vehicle Following/Define Desired Distance ==
  extraSpaceFlag : Inport
  Constant : Constant  Value=h
  Constant1 : Constant  Value=d0
  Constant2 : Constant  Value=hLC
  Constant3 : Constant  Value=d0LC
  Demux : Demux  Outputs=2
  Integrator : Integrator  InitialCondition=[h d0]
  Mux : Mux  Inputs=2
  Mux1 : Mux  Inputs=2
  Saturation1 : Saturate  UpperLimit=hFilterSaturation/2  LowerLimit=-hFilterSaturation
  Sum5 : Sum  Inputs=|+-
  Switch : Switch  Criteria=u2 > Threshold
  hFilterGain : Gain  Gain=hFilterGain
  h : Outport
  d0 : Outport  Port=2
  wires:
  Mux/1 -> Switch/3
  Constant/1 -> Mux/1
  hFilterGain/1 -> Saturation1/1
  Constant2/1 -> Mux1/1
  Sum5/1 -> hFilterGain/1
  Mux1/1 -> Switch/1
  Switch/1 -> Sum5/1
  Constant3/1 -> Mux1/2
  Constant1/1 -> Mux/2
  extraSpaceFlag/1 -> Switch/2
  Saturation1/1 -> Integrator/1
  Integrator/1 -> Demux/1, Sum5/2
  Demux/1 -> h/1
  Demux/2 -> d0/1

== system full_maneuver_single_veh/Fd/Regular Vehicle Following/Veh Following ==
  errors : Inport
  errorsDot : Inport  Port=2
  realInput : Inport  Port=3
  leaderChange : Inport  Port=4
  inRange : Inport  Port=5
  Demux : Demux  Outputs=2
  Demux1 : Demux  Outputs=2
  Gain : Gain  Gain=Ka
  Gain1 : Gain  Gain=Kdd
  Gain3 : Gain  Commented=on  Gain=10
  Integrator1 : Integrator  Commented=on  ExternalReset=either  InitialConditionSource=external  InitialCondition=vx0
  Kd : Gain  Gain=Kd
  Kp : Gain  Gain=Kp
  Saturation : Saturate  Commented=on  UpperLimit=maxComfAccel  LowerLimit=minAcceleration
  Saturation1 : Saturate  UpperLimit=maxGapError  LowerLimit=minGapError
  Scope : Scope  NumInputPorts=6
  Sum : Sum  Inputs=+-|
  Sum1 : Sum  Inputs=+++++
  Sum8 : Sum  Commented=on  Inputs=|+-
  Transport Delay : TransportDelay  DelayTime=0.1
  integralTerm : Subsystem
  u : Outport  VectorParamsAs1DForOutWhenUnconnected=off
  wires:
  inRange/1 -> integralTerm/Enable, Integrator1/2
  Kp/1 -> Sum1/2, Scope/2
  Gain3/1 -> Saturation/1
  Sum8/1 -> Gain3/1
  Saturation/1 -> Integrator1/1
  Integrator1/1 -> Sum8/2
  errors/1 -> Demux/1
  Saturation1/1 -> integralTerm/1(eh), Kp/1
  Demux/2 -> Kd/1  "ev"
  Kd/1 -> Sum1/3, Scope/3
  Demux/1 -> Saturation1/1  "eg"
  leaderChange/1 -> integralTerm/3(leaderChange)
  Transport Delay/1 -> Sum1/1, Scope/1
  realInput/1 -> Sum/2, Integrator1/3
  Sum/1 -> integralTerm/2(inputDiff)
  integralTerm/1(Out1) -> Transport Delay/1
  Gain1/1 -> Sum1/4, Scope/4
  Gain/1 -> Sum1/5, Scope/5
  Sum1/1 -> Sum8/1, Sum/1, Scope/6, u/1
  errorsDot/1 -> Demux1/1
  Demux1/1 -> Gain1/1  "egDot"
  Demux1/2 -> Gain/1  "evDot"

== system full_maneuver_single_veh/Fd/Regular Vehicle Following/Velocity Control ==
  ev : Inport
  ea : Inport  Port=2
  realInput : Inport  Port=3
  Abs : Abs
  Compare To Constant : simulink/Logic and Bit Operations/Compare To Constant  relop=<=  const=0.2  OutDataTypeStr=boolean
  Gain : Gain  Gain=velKd
  Scope : Scope  NumInputPorts=4
  Sum1 : Sum  Inputs=|-+
  Sum3 : Sum  Inputs=+++
  Transport Delay : TransportDelay  DelayTime=0.1
  integral term : Subsystem
  velKp : Gain  Gain=velKp
  u : Outport  VectorParamsAs1DForOutWhenUnconnected=off
  wires:
  Sum3/1 -> Transport Delay/1, Scope/4, u/1
  Gain/1 -> Sum3/3, Scope/3
  ea/1 -> Gain/1
  realInput/1 -> Sum1/1
  velKp/1 -> Sum3/2, Scope/2
  ev/1 -> integral term/1(ev), velKp/1
  Sum1/1 -> Abs/1
  Abs/1 -> Compare To Constant/1
  integral term/1(Out1) -> Scope/1, Sum3/1
  Compare To Constant/1 -> integral term/Enable
  Transport Delay/1 -> Sum1/2

== system full_maneuver_single_veh/Fd/Regular Vehicle Following/Velocity Error ==
  ego : Inport
  velRef : Inport  Port=2
  filterReset : Inport  Port=3
  Bus Selector : BusSelector  OutputSignals=Xdot,xddot
  Gain : Gain  Gain=-1
  Gain3 : Gain  Gain=velFilterGain
  Integrator1 : Integrator  ExternalReset=rising  InitialCondition=vx0
  NOT : Logic  Operator=NOT  IconShape=distinctive  AllPortsSameDT=off  OutDataTypeStr=boolean
  Saturation : Saturate  UpperLimit=maxComfAccel  LowerLimit=minComfAccel
  Sum : Sum  Inputs=+-|
  Sum8 : Sum  Inputs=|+-
  ev : Outport
  ea : Outport  Port=2
  wires:
  NOT/1 -> Integrator1/2
  filterReset/1 -> NOT/1
  Gain/1 -> ea/1
  Sum/1 -> ev/1
  Bus Selector/2 -> Gain/1  "<xddot>"
  Bus Selector/1 -> Sum/2  "<Xdot>"
  ego/1 -> Bus Selector/1
  Integrator1/1 -> Sum8/2, Sum/1
  velRef/1 -> Sum8/1
  Saturation/1 -> Integrator1/1
  Gain3/1 -> Saturation/1
  Sum8/1 -> Gain3/1

== system full_maneuver_single_veh/Fd/Regular Vehicle Following/switch free flow ==
  errors : Inport
  errorsDot : Inport  Port=2
  gap : Inport  Port=3
  h : Inport  Port=4
  d0 : Inport  Port=5
  vRef : Inport  Port=6
  Demux1 : Demux  Outputs=2
  Gain1 : Gain
  MATLAB Function : MATLAB Function  TreatAsAtomicUnit=on
  Relay : Relay  OnSwitchValue=1  OffSwitchValue=-1
  Scope : Scope  NumInputPorts=2
  Selector : Selector  InputPortWidth=2  IndexOptions=Index vector (dialog)  Indices=[2]  OutputSizes=1
  Sum2 : Sum  Inputs=-+
  inRange : Outport  VectorParamsAs1DForOutWhenUnconnected=off
  wires:
  d0/1 -> MATLAB Function/2(d0)
  vRef/1 -> MATLAB Function/3(vRef)
  h/1 -> Gain1/1
  errors/1 -> Selector/1
  gap/1 -> Scope/1, Sum2/1
  Sum2/1 -> Relay/1
  Selector/1 -> MATLAB Function/4(ev)
  Relay/1 -> inRange/1
  Gain1/1 -> MATLAB Function/1(h)
  MATLAB Function/1(maxGap) -> Scope/2, Sum2/2
  errorsDot/1 -> Demux1/1
  Demux1/1 -> MATLAB Function/5(ehDot)
  Demux1/2 -> MATLAB Function/6(ea)

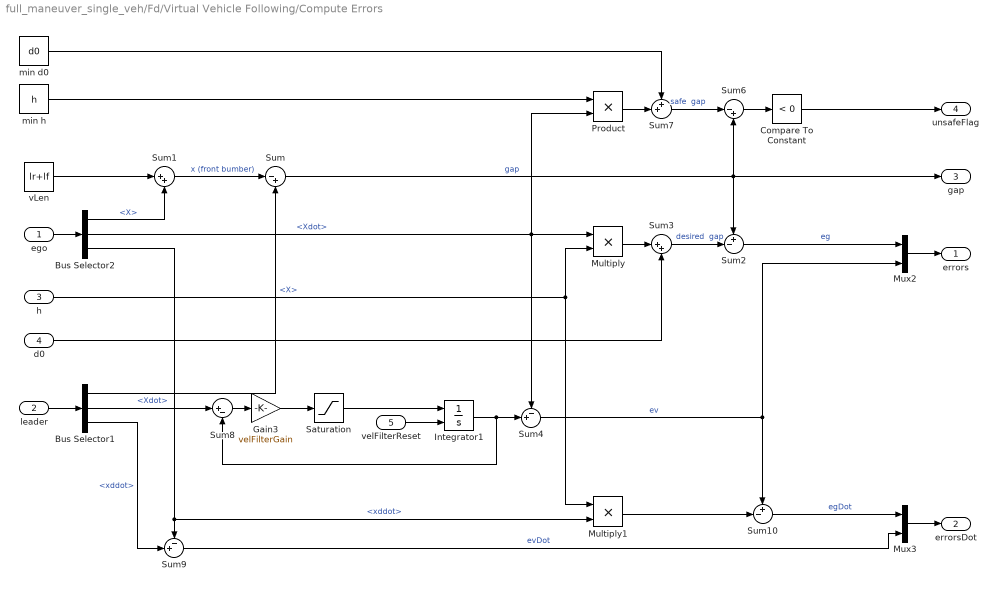
== system full_maneuver_single_veh/Fd/Virtual Vehicle Following/Compute Errors ==
  ego : Inport
  leader : Inport  Port=2
  h : Inport  Port=3
  d0 : Inport  Port=4
  velFilterReset : Inport  Port=5
  Bus Selector1 : BusSelector  OutputSignals=X,Xdot,xddot
  Bus Selector2 : BusSelector  OutputSignals=X,Xdot,xddot
  Compare To Constant : simulink/Logic and Bit Operations/Compare To Constant  relop=<  const=0  OutDataTypeStr=boolean
  Gain3 : Gain  Gain=velFilterGain
  Integrator1 : Integrator  ExternalReset=rising  InitialCondition=vx0
  Multiply : Product
  Multiply1 : Product
  Mux2 : Mux  Inputs=2
  Mux3 : Mux  Inputs=2
  Product : Product
  Saturation : Saturate  UpperLimit=maxAcceleration  LowerLimit=minAcceleration
  Sum : Sum  Inputs=|-+
  Sum1 : Sum  Inputs=|++
  Sum10 : Sum  Inputs=+-|
  Sum2 : Sum  Inputs=+-|
  Sum3 : Sum  Inputs=|++
  Sum4 : Sum  Inputs=-+|
  Sum6 : Sum  Inputs=|-+
  Sum7 : Sum  Inputs=++|
  Sum8 : Sum  Inputs=|+-
  Sum9 : Sum  Inputs=-+|
  min d0 : Constant  Value=d0
  min h : Constant  Value=h
  vLen : Constant  Value=lr+lf
  errors : Outport  VectorParamsAs1DForOutWhenUnconnected=off
  errorsDot : Outport  Port=2
  "gap " : Outport  Port=3  VectorParamsAs1DForOutWhenUnconnected=off
  unsafeFlag : Outport  Port=4  VectorParamsAs1DForOutWhenUnconnected=off
  wires:
  Mux2/1 -> errors/1
  velFilterReset/1 -> Integrator1/2
  Sum6/1 -> Compare To Constant/1
  Sum7/1 -> Sum6/1  "safe  gap"
  min h/1 -> Product/1
  Compare To Constant/1 -> unsafeFlag/1
  Sum2/1 -> Mux2/1  "eg"
  Bus Selector1/1 -> Sum/2  "<X>"
  Product/1 -> Sum7/2
  Sum3/1 -> Sum2/2  "desired  gap"
  Sum1/1 -> Sum/1  "x (front bumber)"
  Bus Selector2/2 -> Sum4/1, Multiply/1, Product/2  "<Xdot>"
  d0/1 -> Sum3/2
  vLen/1 -> Sum1/1
  min d0/1 -> Sum7/1
  Multiply/1 -> Sum3/1
  Sum/1 -> Sum2/1, "gap "/1, Sum6/2  "gap"
  Bus Selector2/1 -> Sum1/2  "<X>"
  h/1 -> Multiply/2, Multiply1/1
  Bus Selector1/2 -> Sum8/1  "<Xdot>"
  Sum4/1 -> Mux2/2, Sum10/1  "ev"
  Gain3/1 -> Saturation/1
  Saturation/1 -> Integrator1/1
  Integrator1/1 -> Sum4/2, Sum8/2
  Sum8/1 -> Gain3/1
  Bus Selector1/3 -> Sum9/2  "<xddot>"
  Bus Selector2/3 -> Sum9/1, Multiply1/2  "<xddot>"
  Multiply1/1 -> Sum10/2
  Sum10/1 -> Mux3/1  "egDot"
  Sum9/1 -> Mux3/2  "evDot"
  Mux3/1 -> errorsDot/1
  ego/1 -> Bus Selector2/1
  leader/1 -> Bus Selector1/1

== system full_maneuver_single_veh/Fd/Virtual Vehicle Following/Define Desired Distance ==
  extraSpaceFlag : Inport
  Constant : Constant  Value=h
  Constant1 : Constant  Value=d0
  Constant2 : Constant  Value=hLC
  Constant3 : Constant  Value=d0LC
  Demux : Demux  Outputs=2
  Integrator : Integrator  InitialCondition=[h d0]
  Mux : Mux  Inputs=2
  Mux1 : Mux  Inputs=2
  Saturation1 : Saturate  UpperLimit=hFilterSaturation/2  LowerLimit=-hFilterSaturation
  Sum5 : Sum  Inputs=|+-
  Switch : Switch  Criteria=u2 > Threshold
  hFilterGain : Gain  Gain=hFilterGain
  h : Outport
  d0 : Outport  Port=2
  wires:
  Mux/1 -> Switch/3
  Constant/1 -> Mux/1
  hFilterGain/1 -> Saturation1/1
  Constant2/1 -> Mux1/1
  Sum5/1 -> hFilterGain/1
  Mux1/1 -> Switch/1
  Switch/1 -> Sum5/1
  Constant3/1 -> Mux1/2
  Constant1/1 -> Mux/2
  extraSpaceFlag/1 -> Switch/2
  Saturation1/1 -> Integrator/1
  Integrator/1 -> Demux/1, Sum5/2
  Demux/1 -> h/1
  Demux/2 -> d0/1
